simulink model "BFE_TestHarness"  (Simulink 8.6)
settings: Solver=FixedStepDiscrete  StartTime=0.0  StopTime=3  FixedStep=Ts  RelTol=1e-3
PreLoadFcn:
  | addpath('MBD_Tests')
  | 
  | load('Workspace\EnvVar.mat')
  | run('MBD_Tests\MBD_tests_init.m')
  | if exist('tl_preloadfcn','file'), tl_preloadfcn(gcs,402); end
PostLoadFcn:
  | if exist('tl_postloadfcn','file'), tl_postloadfcn(gcs,402); end
InitFcn:
  | if exist('tlds_init','file'), tlds_init(gcs); end
StartFcn:
  | if exist('tlds_start','file'), tlds_start(gcs); end
StopFcn:
  | if exist('tlds_stop','file'), tlds_stop(gcs); end
undefined symbols (not defined in the file): ddv, Ts, u2, u3, u4
libraries: tllib x11, simulink x8, LIB_TF_G_111 x2, LIB_TF_G_12_StepControl x2, LIB_TF_G_112 x1, LIB_TF_G_113 x1
(part 6 of 17)

== system BFE_TestHarness/BFE_AC_BeltFunctionExecution/Subsystem/BFE_AC_BeltFunctionExecution/BFE_AC_BeltFunctionExecution/BFE_runExecuteStandardSteps/ExecuteStandardSteps/SubsystemUpdateConsigns ==
  lMilliOrderIncrement : Inport  RequirementInfo={} %GIDa_5cc21bd3_cc40_44a3_8bbb_1525dfc2aeeb
  lMilliOrder : Inport  RequirementInfo={} %GIDa_1a8363d0_9cc4_4d0f_87bb_7cd28cf3fc20  Port=2
  Add : Sum  RequirementInfo={} %GIDa_7faf4d1b_26d0_400a_863a_5a4ca9203508  SaturateOnIntegerOverflow=on  mask(TL_Sum){data={'output',{'name','s32UpdTargetStepOnGoing','type','Int32','checkmin',1,'checkmax',1},'date',735951.66850537038}}
      settings: CopyFcn=if exist('tl_reset_reviewflag','file')==2,tl_reset_reviewflag(gcbh);end  DeleteFcn=if exist('delete_tlblock','file')==2,delete_tlblock(gcbh);end  NameChangeFcn=if exist('rename_tlblock','file')==2,rename_tlblock(gcbh);end  OpenFcn=if exist('tl_open_blockdlg','file')==2,tl_open_blockdlg(gcbh);else,open_system(gcbh,'parameter');end
      mask Help: eval(['if exist(''tl_online_help'',''file'') == 2, tl_online_help(''Topic'',''TL_Sum''),else, web([''jar:file:///'',matlabroot,''/help/toolbox/simulink/help.jar!/slref/' lower(get_param(gcbh,'Blocktype')) '.html''], ''-helpbrowser''),end'])
      mask Display: plot([-0.05, 1.05, NaN, -0.05, 1.05],[.01, .01, NaN, .99, .99])
  Add1 : Sum  RequirementInfo={} %GIDa_66a69bfa_962f_4ea5_a228_a0bc3a3f5b5e  SaturateOnIntegerOverflow=on  mask(TL_Sum){data={'output',{'name','s32UpdTargetStartStep','type','Int32','checkmin',1,'checkmax',1},'date',735951.66850499995}}
      settings: CopyFcn=if exist('tl_reset_reviewflag','file')==2,tl_reset_reviewflag(gcbh);end  DeleteFcn=if exist('delete_tlblock','file')==2,delete_tlblock(gcbh);end  NameChangeFcn=if exist('rename_tlblock','file')==2,rename_tlblock(gcbh);end  OpenFcn=if exist('tl_open_blockdlg','file')==2,tl_open_blockdlg(gcbh);else,open_system(gcbh,'parameter');end
      mask Help: eval(['if exist(''tl_online_help'',''file'') == 2, tl_online_help(''Topic'',''TL_Sum''),else, web([''jar:file:///'',matlabroot,''/help/toolbox/simulink/help.jar!/slref/' lower(get_param(gcbh,'Blocktype')) '.html''], ''-helpbrowser''),end'])
      mask Display: plot([-0.05, 1.05, NaN, -0.05, 1.05],[.01, .01, NaN, .99, .99])
  SubsystemDetectConsignsChange : Subsystem  RequirementInfo={} %GIDa_913f49ce_43de_40fd_b174_3a8dea1fc7ca
  Switch : Switch  RequirementInfo={} %GIDa_e7269de4_dc33_4d7b_91a9_ffc23af86bd1  Criteria=u2 ~= 0  mask(TL_Switch){data={'output',{'name','s32StepTarget2ms','inheritscaling',1},'threshold',{'scalar',1},'date',735951.66850278934}}
      settings: CopyFcn=if exist('tl_reset_reviewflag','file')==2,tl_reset_reviewflag(gcbh);end  DeleteFcn=if exist('delete_tlblock','file')==2,delete_tlblock(gcbh);end  NameChangeFcn=if exist('rename_tlblock','file')==2,rename_tlblock(gcbh);end  OpenFcn=if exist('tl_open_blockdlg','file')==2,tl_open_blockdlg(gcbh);else,open_system(gcbh,'parameter');end
      mask Help: eval(['if exist(''tl_online_help'',''file'') == 2, tl_online_help(''Topic'',''TL_Switch''),else, web([''jar:file:///'',matlabroot,''/help/toolbox/simulink/help.jar!/slref/' lower(get_param(gcbh,'Blocktype')) '.html''], ''-helpbrowser''),end'])
      mask Display: plot([-0.05, 1.05, NaN, -0.05, 1.05],[.01, .01, NaN, .99, .99])
  Unit Delay : UnitDelay  RequirementInfo={} %GIDa_e30283f1_fb3e_4a2a_b6d4_05ae56e450b9  SampleTime=-1  mask(TL_UnitDelay){data={'output',{'type','Int32'},'state',{'name','s32PrevStepTarget2ms','type','Int32'},'date',735951.66850224533}}
      settings: CopyFcn=if exist('tl_reset_reviewflag','file')==2,tl_reset_reviewflag(gcbh);end  DeleteFcn=if exist('delete_tlblock','file')==2,delete_tlblock(gcbh);end  NameChangeFcn=if exist('rename_tlblock','file')==2,rename_tlblock(gcbh);end  OpenFcn=if exist('tl_open_blockdlg','file')==2,tl_open_blockdlg(gcbh);else,open_system(gcbh,'parameter');end
      mask Help: eval(['if exist(''tl_online_help'',''file'') == 2, tl_online_help(''Topic'',''TL_UnitDelay''),else, web([''jar:file:///'',matlabroot,''/help/toolbox/simulink/help.jar!/slref/' lower(get_param(gcbh,'Blocktype')) '.html''], ''-helpbrowser''),end'])
      mask Display: plot([-0.05, 1.05, NaN, -0.05, 1.05],[.01, .01, NaN, .99, .99])
  bAreConsignsChanged : Outport  RequirementInfo={} %GIDa_218da950_518a_4cec_bd68_380cd2445e8d
  lOrderToApply : Outport  RequirementInfo={} %GIDa_afcc631f_1aa7_4131_a13d_9b5c398a8bc9  Port=2
  wires:
  Add1/1 -> Switch/1
  Unit Delay/1 -> Add/2
  Add/1 -> Switch/3
  Switch/1 -> Unit Delay/1, lOrderToApply/1
  SubsystemDetectConsignsChange/1(bAreConsignsChanged_out) -> bAreConsignsChanged/1, Switch/2
  lMilliOrder/1 -> Add1/1, SubsystemDetectConsignsChange/1(lFirstOrder)
  lMilliOrderIncrement/1 -> Add1/2, Add/1, SubsystemDetectConsignsChange/2(lIncrement)

== system BFE_TestHarness/BFE_AC_BeltFunctionExecution/Subsystem/BFE_AC_BeltFunctionExecution/BFE_AC_BeltFunctionExecution/BFE_runScheduleStep/Critical section for outputs to  protect against ISR access/Switch Case Action Subsystem ==
  In1 : Inport
  Trigger : TriggerPort  TriggerType=function-call
  s32OrderIncrementValue : Outport  PortDimensions=1  mask(TL_Outport){data={'autosar',{'useautosarcommunication',1,'kind',3,'communicationmode',1,'interrunnablevariable','s32OrderIncrementValue'},'date',736809.44014983799}}
      settings: CopyFcn=if exist('tl_reset_reviewflag','file')==2,tl_reset_reviewflag(gcbh);end  DeleteFcn=if exist('delete_tlblock','file')==2,delete_tlblock(gcbh);end  NameChangeFcn=if exist('rename_tlblock','file')==2,rename_tlblock(gcbh);end  OpenFcn=if exist('tl_open_blockdlg','file')==2,tl_open_blockdlg(gcbh);else,open_system(gcbh,'parameter');end
      mask Help: eval(['if exist(''tl_online_help'',''file'') == 2, tl_online_help(''Topic'',''TL_Outport''),else, web([''jar:file:///'',matlabroot,''/help/toolbox/simulink/help.jar!/slref/' lower(get_param(gcbh,'Blocktype')) '.html''], ''-helpbrowser''),end'])
      mask Display: plot([0.2 0.35 NaN 0.65 0.8],[0 1 NaN 0 1]);
  wires:
  In1/1 -> s32OrderIncrementValue/1

== system BFE_TestHarness/BFE_AC_BeltFunctionExecution/Subsystem/BFE_AC_BeltFunctionExecution/BFE_AC_BeltFunctionExecution/BFE_runScheduleStep/Critical section for outputs to  protect against ISR access/Switch Case Action Subsystem1 ==
  In1 : Inport
  Trigger : TriggerPort  TriggerType=function-call
  s32FirstOrderValue : Outport  PortDimensions=1  mask(TL_Outport){data={'autosar',{'useautosarcommunication',1,'kind',3,'communicationmode',1,'interrunnablevariable','s32FirstOrderValue'},'date',736809.44014995371}}
      settings: CopyFcn=if exist('tl_reset_reviewflag','file')==2,tl_reset_reviewflag(gcbh);end  DeleteFcn=if exist('delete_tlblock','file')==2,delete_tlblock(gcbh);end  NameChangeFcn=if exist('rename_tlblock','file')==2,rename_tlblock(gcbh);end  OpenFcn=if exist('tl_open_blockdlg','file')==2,tl_open_blockdlg(gcbh);else,open_system(gcbh,'parameter');end
      mask Help: eval(['if exist(''tl_online_help'',''file'') == 2, tl_online_help(''Topic'',''TL_Outport''),else, web([''jar:file:///'',matlabroot,''/help/toolbox/simulink/help.jar!/slref/' lower(get_param(gcbh,'Blocktype')) '.html''], ''-helpbrowser''),end'])
      mask Display: plot([0.2 0.35 NaN 0.65 0.8],[0 1 NaN 0 1]);
  wires:
  In1/1 -> s32FirstOrderValue/1

== system BFE_TestHarness/BFE_AC_BeltFunctionExecution/Subsystem/BFE_AC_BeltFunctionExecution/BFE_AC_BeltFunctionExecution/BFE_runScheduleStep/Critical section for outputs to  protect against ISR access/Switch Case Action Subsystem2 ==
  In1 : Inport
  Trigger : TriggerPort  TriggerType=function-call
  u16StepDuration : Outport  PortDimensions=1  mask(TL_Outport){data={'autosar',{'useautosarcommunication',1,'kind',3,'communicationmode',1,'interrunnablevariable','u16StepDuration'},'date',736809.44015006942}}
      settings: CopyFcn=if exist('tl_reset_reviewflag','file')==2,tl_reset_reviewflag(gcbh);end  DeleteFcn=if exist('delete_tlblock','file')==2,delete_tlblock(gcbh);end  NameChangeFcn=if exist('rename_tlblock','file')==2,rename_tlblock(gcbh);end  OpenFcn=if exist('tl_open_blockdlg','file')==2,tl_open_blockdlg(gcbh);else,open_system(gcbh,'parameter');end
      mask Help: eval(['if exist(''tl_online_help'',''file'') == 2, tl_online_help(''Topic'',''TL_Outport''),else, web([''jar:file:///'',matlabroot,''/help/toolbox/simulink/help.jar!/slref/' lower(get_param(gcbh,'Blocktype')) '.html''], ''-helpbrowser''),end'])
      mask Display: plot([0.2 0.35 NaN 0.65 0.8],[0 1 NaN 0 1]);
  wires:
  In1/1 -> u16StepDuration/1

== system BFE_TestHarness/BFE_AC_BeltFunctionExecution/Subsystem/BFE_AC_BeltFunctionExecution/BFE_AC_BeltFunctionExecution/BFE_runScheduleStep/Critical section for outputs to  protect against ISR access/Switch Case Action Subsystem3 ==
  In1 : Inport
  Trigger : TriggerPort  TriggerType=function-call
  u8OrderType : Outport  PortDimensions=1  mask(TL_Outport){data={'autosar',{'useautosarcommunication',1,'kind',3,'communicationmode',1,'interrunnablevariable','u8OrderType'},'date',736809.44015030097}}
      settings: CopyFcn=if exist('tl_reset_reviewflag','file')==2,tl_reset_reviewflag(gcbh);end  DeleteFcn=if exist('delete_tlblock','file')==2,delete_tlblock(gcbh);end  NameChangeFcn=if exist('rename_tlblock','file')==2,rename_tlblock(gcbh);end  OpenFcn=if exist('tl_open_blockdlg','file')==2,tl_open_blockdlg(gcbh);else,open_system(gcbh,'parameter');end
      mask Help: eval(['if exist(''tl_online_help'',''file'') == 2, tl_online_help(''Topic'',''TL_Outport''),else, web([''jar:file:///'',matlabroot,''/help/toolbox/simulink/help.jar!/slref/' lower(get_param(gcbh,'Blocktype')) '.html''], ''-helpbrowser''),end'])
      mask Display: plot([0.2 0.35 NaN 0.65 0.8],[0 1 NaN 0 1]);
  wires:
  In1/1 -> u8OrderType/1

== system BFE_TestHarness/BFE_AC_BeltFunctionExecution/Subsystem/BFE_AC_BeltFunctionExecution/BFE_AC_BeltFunctionExecution/ManageRunnables/If Action Subsystem/If Action Subsystem ==
  Action Port : ActionPort  RequirementInfo={} %GIDa_a62ee4e6_0f79_4252_9fe2_412ab995a6fd  ActionType=then
  Function-Call Generator : simulink/Ports & Subsystems/Function-Call Generator  RequirementInfo={} %GIDa_58f86ece_75e2_4389_8d97_59eeed75d555  sample_time=-1  numberOfIterations=1
  Out1 : Outport  RequirementInfo={} %GIDa_7be6b692_a524_497d_b672_83760d64e461
  wires:
  Function-Call Generator/1 -> Out1/1

== system BFE_TestHarness/BFE_AC_BeltFunctionExecution/Subsystem/BFE_AC_BeltFunctionExecution/BFE_AC_BeltFunctionExecution/ManageRunnables/If Action Subsystem1/If Action Subsystem ==
  Action Port : ActionPort  RequirementInfo={} %GIDa_89bb6ac8_18ae_4522_a67e_c5de92d9804a  ActionType=then
  Function-Call Generator : simulink/Ports & Subsystems/Function-Call Generator  RequirementInfo={} %GIDa_4ed9d91c_f3a7_4384_b10d_86c6c5719deb  sample_time=-1  numberOfIterations=1
  Out1 : Outport  RequirementInfo={} %GIDa_e16df5b7_c629_412d_97e3_521d5db63317
  wires:
  Function-Call Generator/1 -> Out1/1

== system BFE_TestHarness/BFE_AC_BeltFunctionExecution/Subsystem/BFE_AC_BeltFunctionExecution/BFE_AC_BeltFunctionExecution/ManageRunnables/If Action Subsystem2/If Action Subsystem1 ==
  Action Port : ActionPort  RequirementInfo={} %GIDa_29c84838_766b_4990_bc41_364801b2a2c1  ActionType=then
  Function-Call Generator : simulink/Ports & Subsystems/Function-Call Generator  RequirementInfo={} %GIDa_00d024fe_ccfb_4152_8998_5dbb5a8dc91c  sample_time=-1  numberOfIterations=1
  Out1 : Outport  RequirementInfo={} %GIDa_21bb2b30_61bd_4376_a26f_0f487527c63e
  wires:
  Function-Call Generator/1 -> Out1/1

== system BFE_TestHarness/BFE_AC_BeltFunctionExecution/Subsystem/BFE_AC_BeltFunctionExecution/BFE_AC_BeltFunctionExecution/ManageRunnables/If Action Subsystem2/If Action Subsystem2 ==
  Action Port : ActionPort  RequirementInfo={} %GIDa_7511eba7_1284_477b_a038_8ef99bfcc2bb  ActionType=else
  Function-Call Generator : simulink/Ports & Subsystems/Function-Call Generator  RequirementInfo={} %GIDa_1326366b_347a_4b1b_b860_6f0899239335  sample_time=-1  numberOfIterations=1
  Out1 : Outport  RequirementInfo={} %GIDa_86f1c9bb_def5_449e_be28_356b79e30475
  wires:
  Function-Call Generator/1 -> Out1/1

== system BFE_TestHarness/BFE_AC_BeltFunctionExecution/Subsystem/BFE_AC_BeltFunctionExecution/BFE_AC_BeltFunctionExecution/ManageRunnables/If Action Subsystem3/If Action Subsystem1 ==
  Action Port : ActionPort  RequirementInfo={} %GIDa_99ef5362_0467_4fc1_9784_994714b2c9a7  ActionType=then
  Function-Call Generator : simulink/Ports & Subsystems/Function-Call Generator  RequirementInfo={} %GIDa_c0aab7a0_dc5d_4927_bcec_735c68472a75  sample_time=-1  numberOfIterations=1
  Out1 : Outport  RequirementInfo={} %GIDa_15a0167e_97c9_4a94_b857_ffa23d77dc58
  wires:
  Function-Call Generator/1 -> Out1/1

== system BFE_TestHarness/BFE_AC_BeltFunctionExecution/Subsystem/BFE_AC_BeltFunctionExecution/BFE_AC_BeltFunctionExecution/BFE_runExecuteHighPowerStep/HP feature activated/CurrentRegulation/BoostInterruptConditions_MotorCurrent ==
  note: If the duty cycle of the PWM for the boost is maximum and if the current is too weak, the boost is interrupted (the value of the duty cycle is decreased)
  s16Current : Inport  RequirementInfo={} %GIDa_fed87945_4a58_47d6_bead_1101b99165da
  s16Integer : Inport  RequirementInfo={} %GIDa_19139cd3_6afd_4d73_a336_46a3cf0ace48  Port=2
  s16IntegerMax : Inport  RequirementInfo={} %GIDa_a1f576fc_1114_4384_8991_b2635a757868  Port=3
  KU8_MIN_CURRENT_DURING_BOOST : Constant  RequirementInfo={} %GIDa_fe38ee79_2149_41c8_8830_b3ef7000511c  Value=ddv('BFE_Config_Data/KU8_MIN_CURRENT_DURING_BOOST')  mask(TL_Constant){data={'output',{'variable','BFE_Config_Data/KU8_MIN_CURRENT_DURING_BOOST'},'date',735951.6685871759}}
      settings: CopyFcn=if exist('tl_reset_reviewflag','file')==2,tl_reset_reviewflag(gcbh);end  DeleteFcn=if exist('delete_tlblock','file')==2,delete_tlblock(gcbh);end  NameChangeFcn=if exist('rename_tlblock','file')==2,rename_tlblock(gcbh);end  OpenFcn=if exist('tl_open_blockdlg','file')==2,tl_open_blockdlg(gcbh);else,open_system(gcbh,'parameter');end
      mask Help: eval(['if exist(''tl_online_help'',''file'') == 2, tl_online_help(''Topic'',''TL_Constant''),else, web([''jar:file:///'',matlabroot,''/help/toolbox/simulink/help.jar!/slref/' lower(get_param(gcbh,'Blocktype')) '.html''], ''-helpbrowser''),end'])
      mask Display: plot([-0.05, 1.05, NaN, -0.05, 1.05],[.01, .01, NaN, .99, .99])
  Logical Operator1 : Logic  RequirementInfo={} %GIDa_242a9706_3112_44f3_83e7_a7f476e04a26  AllPortsSameDT=off  OutDataTypeStr=boolean  mask(TL_LogicalOperator){data={'output',{'name','bBoostInterrupt'},'date',735951.66858680558}}
      settings: DeleteFcn=if exist('delete_tlblock','file')==2,delete_tlblock(gcbh);end  NameChangeFcn=if exist('rename_tlblock','file')==2,rename_tlblock(gcbh);end  OpenFcn=if exist('tl_open_blockdlg','file')==2,tl_open_blockdlg(gcbh);else,open_system(gcbh,'parameter');end
      mask Help: eval(['if exist(''tl_online_help'',''file'') == 2, tl_online_help(''Topic'',''TL_LogicalOperator''),else, web([''jar:file:///'',matlabroot,''/help/toolbox/simulink/help.jar!/slref/' lower(get_param(gcbh,'Blocktype')) '.html''], ''-helpbrowser''),end'])
      mask Display: plot([-0.05, 1.05, NaN, -0.05, 1.05],[.01, .01, NaN, .99, .99])
  Relational Operator : RelationalOperator  RequirementInfo={} %GIDa_2bfdd7ae_5bd4_46be_b807_9ae38a2e5e84  OutDataTypeStr=boolean  mask(TL_RelationalOperator){data={'date',735951.66858653934}}
      settings: DeleteFcn=if exist('delete_tlblock','file')==2,delete_tlblock(gcbh);end  NameChangeFcn=if exist('rename_tlblock','file')==2,rename_tlblock(gcbh);end  OpenFcn=if exist('tl_open_blockdlg','file')==2,tl_open_blockdlg(gcbh);else,open_system(gcbh,'parameter');end
      mask Help: eval(['if exist(''tl_online_help'',''file'') == 2, tl_online_help(''Topic'',''TL_RelationalOperator''),else, web([''jar:file:///'',matlabroot,''/help/toolbox/simulink/help.jar!/slref/' lower(get_param(gcbh,'Blocktype')) '.html''], ''-helpbrowser''),end'])
      mask Display: plot([-0.05, 1.05, NaN, -0.05, 1.05],[.01, .01, NaN, .99, .99])
  Relational Operator1 : RelationalOperator  RequirementInfo={} %GIDa_3d94211e_eea3_4510_ab5c_091b41b511c7  Operator=<  OutDataTypeStr=boolean  mask(TL_RelationalOperator){data={'date',735951.66858628474}}
      settings: DeleteFcn=if exist('delete_tlblock','file')==2,delete_tlblock(gcbh);end  NameChangeFcn=if exist('rename_tlblock','file')==2,rename_tlblock(gcbh);end  OpenFcn=if exist('tl_open_blockdlg','file')==2,tl_open_blockdlg(gcbh);else,open_system(gcbh,'parameter');end
      mask Help: eval(['if exist(''tl_online_help'',''file'') == 2, tl_online_help(''Topic'',''TL_RelationalOperator''),else, web([''jar:file:///'',matlabroot,''/help/toolbox/simulink/help.jar!/slref/' lower(get_param(gcbh,'Blocktype')) '.html''], ''-helpbrowser''),end'])
      mask Display: plot([-0.05, 1.05, NaN, -0.05, 1.05],[.01, .01, NaN, .99, .99])
  bBoostInterrupt : Outport  RequirementInfo={} %GIDa_c813631b_598e_4f6c_b47e_8999c2167893
  wires:
  Relational Operator/1 -> Logical Operator1/2
  KU8_MIN_CURRENT_DURING_BOOST/1 -> Relational Operator1/2
  Relational Operator1/1 -> Logical Operator1/1
  s16Current/1 -> Relational Operator1/1
  s16Integer/1 -> Relational Operator/1
  s16IntegerMax/1 -> Relational Operator/2
  Logical Operator1/1 -> bBoostInterrupt/1

== system BFE_TestHarness/BFE_AC_BeltFunctionExecution/Subsystem/BFE_AC_BeltFunctionExecution/BFE_AC_BeltFunctionExecution/BFE_runExecuteHighPowerStep/HP feature activated/CurrentRegulation/BoostInterruptConditions_Timing ==
  s16OldInteger : Inport  RequirementInfo={} %GIDa_e89f5e19_b5a3_4ada_b2f7_21fc6d90613f
  bBoostTimeElapsed : Inport  RequirementInfo={} %GIDa_225092f2_0ca9_4ed5_8258_126e03d9d686  Port=2
  KUS_PWM_MAX_BTN : Constant  RequirementInfo={} %GIDa_a70c20e3_f31f_4c1c_a99f_96ca4cd62288  Value=ddv('BFE/KS16_PWM_MAX_BTN')  OutDataTypeStr=uint16  mask(TL_Constant){data={'output',{'variable','BFE/KS16_PWM_MAX_BTN'},'date',735951.66858603014}}
      settings: CopyFcn=if exist('tl_reset_reviewflag','file')==2,tl_reset_reviewflag(gcbh);end  DeleteFcn=if exist('delete_tlblock','file')==2,delete_tlblock(gcbh);end  NameChangeFcn=if exist('rename_tlblock','file')==2,rename_tlblock(gcbh);end  OpenFcn=if exist('tl_open_blockdlg','file')==2,tl_open_blockdlg(gcbh);else,open_system(gcbh,'parameter');end
      mask Help: eval(['if exist(''tl_online_help'',''file'') == 2, tl_online_help(''Topic'',''TL_Constant''),else, web([''jar:file:///'',matlabroot,''/help/toolbox/simulink/help.jar!/slref/' lower(get_param(gcbh,'Blocktype')) '.html''], ''-helpbrowser''),end'])
      mask Display: plot([-0.05, 1.05, NaN, -0.05, 1.05],[.01, .01, NaN, .99, .99])
  Logical Operator1 : Logic  RequirementInfo={} %GIDa_9fd42152_b135_49c9_aa59_88d817c1c9ee  AllPortsSameDT=off  OutDataTypeStr=boolean  mask(TL_LogicalOperator){data={'output',{'name','bStartBoostDecrease'},'date',735951.66858567134}}
      settings: DeleteFcn=if exist('delete_tlblock','file')==2,delete_tlblock(gcbh);end  NameChangeFcn=if exist('rename_tlblock','file')==2,rename_tlblock(gcbh);end  OpenFcn=if exist('tl_open_blockdlg','file')==2,tl_open_blockdlg(gcbh);else,open_system(gcbh,'parameter');end
      mask Help: eval(['if exist(''tl_online_help'',''file'') == 2, tl_online_help(''Topic'',''TL_LogicalOperator''),else, web([''jar:file:///'',matlabroot,''/help/toolbox/simulink/help.jar!/slref/' lower(get_param(gcbh,'Blocktype')) '.html''], ''-helpbrowser''),end'])
      mask Display: plot([-0.05, 1.05, NaN, -0.05, 1.05],[.01, .01, NaN, .99, .99])
  Relational Operator : RelationalOperator  RequirementInfo={} %GIDa_0d852afc_57d9_4a42_8a62_1695fcfafa0b  Operator=>  OutDataTypeStr=boolean  mask(TL_RelationalOperator){data={'output',{'name','bBoostOn'},'date',735951.6685854051}}
      settings: DeleteFcn=if exist('delete_tlblock','file')==2,delete_tlblock(gcbh);end  NameChangeFcn=if exist('rename_tlblock','file')==2,rename_tlblock(gcbh);end  OpenFcn=if exist('tl_open_blockdlg','file')==2,tl_open_blockdlg(gcbh);else,open_system(gcbh,'parameter');end
      mask Help: eval(['if exist(''tl_online_help'',''file'') == 2, tl_online_help(''Topic'',''TL_RelationalOperator''),else, web([''jar:file:///'',matlabroot,''/help/toolbox/simulink/help.jar!/slref/' lower(get_param(gcbh,'Blocktype')) '.html''], ''-helpbrowser''),end'])
      mask Display: plot([-0.05, 1.05, NaN, -0.05, 1.05],[.01, .01, NaN, .99, .99])
  bStartBoostDecrease : Outport  RequirementInfo={} %GIDa_daa43caa_cf1f_47eb_8219_5321a27842ad
  wires:
  Logical Operator1/1 -> bStartBoostDecrease/1
  s16OldInteger/1 -> Relational Operator/1
  KUS_PWM_MAX_BTN/1 -> Relational Operator/2
  bBoostTimeElapsed/1 -> Logical Operator1/1
  Relational Operator/1 -> Logical Operator1/2

== system BFE_TestHarness/BFE_AC_BeltFunctionExecution/Subsystem/BFE_AC_BeltFunctionExecution/BFE_AC_BeltFunctionExecution/BFE_runExecuteHighPowerStep/HP feature activated/CurrentRegulation/CalculateIntegerInit ==
  note: IntegerInit = (6400 * Iorder)/KL30
  s16FirstOrderValue : Inport  RequirementInfo={} %GIDa_c817c6f4_52c0_448f_b6ca_a57fed24fcee
  u16BatteryVoltage : Inport  RequirementInfo={} %GIDa_798de003_9265_4dce_9db6_fac1c754e338  Port=2
  KU16_INIT_INTEGER_GAIN_DEN : Constant  Value=ddv('BFE/KU16_INIT_INTEGER_GAIN_DEN')  OutDataTypeStr=uint16  mask(TL_Constant){data={'output',{'variable','BFE/KU16_INIT_INTEGER_GAIN_DEN'},'date',735951.66858512734}}
      settings: CopyFcn=if exist('tl_reset_reviewflag','file')==2,tl_reset_reviewflag(gcbh);end  DeleteFcn=if exist('delete_tlblock','file')==2,delete_tlblock(gcbh);end  NameChangeFcn=if exist('rename_tlblock','file')==2,rename_tlblock(gcbh);end  OpenFcn=if exist('tl_open_blockdlg','file')==2,tl_open_blockdlg(gcbh);else,open_system(gcbh,'parameter');end
      mask Help: eval(['if exist(''tl_online_help'',''file'') == 2, tl_online_help(''Topic'',''TL_Constant''),else, web([''jar:file:///'',matlabroot,''/help/toolbox/simulink/help.jar!/slref/' lower(get_param(gcbh,'Blocktype')) '.html''], ''-helpbrowser''),end'])
      mask Display: plot([-0.05, 1.05, NaN, -0.05, 1.05],[.01, .01, NaN, .99, .99])
  KU16_INIT_INTEGER_GAIN_NOM : Constant  Value=ddv('BFE/KU16_INIT_INTEGER_GAIN_NOM')  OutDataTypeStr=uint16  mask(TL_Constant){data={'output',{'variable','BFE/KU16_INIT_INTEGER_GAIN_NOM'},'date',735951.66858474538}}
      settings: CopyFcn=if exist('tl_reset_reviewflag','file')==2,tl_reset_reviewflag(gcbh);end  DeleteFcn=if exist('delete_tlblock','file')==2,delete_tlblock(gcbh);end  NameChangeFcn=if exist('rename_tlblock','file')==2,rename_tlblock(gcbh);end  OpenFcn=if exist('tl_open_blockdlg','file')==2,tl_open_blockdlg(gcbh);else,open_system(gcbh,'parameter');end
      mask Help: eval(['if exist(''tl_online_help'',''file'') == 2, tl_online_help(''Topic'',''TL_Constant''),else, web([''jar:file:///'',matlabroot,''/help/toolbox/simulink/help.jar!/slref/' lower(get_param(gcbh,'Blocktype')) '.html''], ''-helpbrowser''),end'])
      mask Display: plot([-0.05, 1.05, NaN, -0.05, 1.05],[.01, .01, NaN, .99, .99])
  KUS_PWM_MAX_BTN : Constant  RequirementInfo={} %GIDa_88135799_6637_44ef_a568_3f4a11047fb4  Value=ddv('BFE/KS16_PWM_MAX_BTN')  OutDataTypeStr=uint16  mask(TL_Constant){data={'output',{'variable','BFE/KS16_PWM_MAX_BTN'},'date',735951.66858435189}}
      settings: CopyFcn=if exist('tl_reset_reviewflag','file')==2,tl_reset_reviewflag(gcbh);end  DeleteFcn=if exist('delete_tlblock','file')==2,delete_tlblock(gcbh);end  NameChangeFcn=if exist('rename_tlblock','file')==2,rename_tlblock(gcbh);end  OpenFcn=if exist('tl_open_blockdlg','file')==2,tl_open_blockdlg(gcbh);else,open_system(gcbh,'parameter');end
      mask Help: eval(['if exist(''tl_online_help'',''file'') == 2, tl_online_help(''Topic'',''TL_Constant''),else, web([''jar:file:///'',matlabroot,''/help/toolbox/simulink/help.jar!/slref/' lower(get_param(gcbh,'Blocktype')) '.html''], ''-helpbrowser''),end'])
      mask Display: plot([-0.05, 1.05, NaN, -0.05, 1.05],[.01, .01, NaN, .99, .99])
  Product1 : Product  RequirementInfo={} %GIDa_5e5e27d2_ccc2_478f_b2ba_8d03c9d029d9  Inputs=**  OutDataTypeStr=uint32  RndMeth=Zero  mask(TL_Product){data={'output',{'type','Int32'},'date',735951.66858395829}}
      settings: CopyFcn=if exist('tl_reset_reviewflag','file')==2,tl_reset_reviewflag(gcbh);end  DeleteFcn=if exist('delete_tlblock','file')==2,delete_tlblock(gcbh);end  NameChangeFcn=if exist('rename_tlblock','file')==2,rename_tlblock(gcbh);end  OpenFcn=if exist('tl_open_blockdlg','file')==2,tl_open_blockdlg(gcbh);else,open_system(gcbh,'parameter');end
      mask Help: eval(['if exist(''tl_online_help'',''file'') == 2, tl_online_help(''Topic'',''TL_Product''),else, web([''jar:file:///'',matlabroot,''/help/toolbox/simulink/help.jar!/slref/' lower(get_param(gcbh,'Blocktype')) '.html''], ''-helpbrowser''),end'])
      mask Display: plot([-0.05, 1.05, NaN, -0.05, 1.05],[.01, .01, NaN, .99, .99])
  Product2 : Product  RequirementInfo={} %GIDa_c96c8a8f_b421_4d94_8a8b_1faf2b26a1c7  Inputs=*/  OutDataTypeStr=uint32  RndMeth=Zero  mask(TL_Product){data={'output',{'name','s16IntegerInit','type','UInt32'},'date',735951.66858358798}}
      settings: CopyFcn=if exist('tl_reset_reviewflag','file')==2,tl_reset_reviewflag(gcbh);end  DeleteFcn=if exist('delete_tlblock','file')==2,delete_tlblock(gcbh);end  NameChangeFcn=if exist('rename_tlblock','file')==2,rename_tlblock(gcbh);end  OpenFcn=if exist('tl_open_blockdlg','file')==2,tl_open_blockdlg(gcbh);else,open_system(gcbh,'parameter');end
      mask Help: eval(['if exist(''tl_online_help'',''file'') == 2, tl_online_help(''Topic'',''TL_Product''),else, web([''jar:file:///'',matlabroot,''/help/toolbox/simulink/help.jar!/slref/' lower(get_param(gcbh,'Blocktype')) '.html''], ''-helpbrowser''),end'])
      mask Display: plot([-0.05, 1.05, NaN, -0.05, 1.05],[.01, .01, NaN, .99, .99])
  Product3 : Product  Inputs=**  OutDataTypeStr=uint32  RndMeth=Zero  mask(TL_Product){data={'output',{'type','UInt32'},'date',735951.66858320602}}
      settings: CopyFcn=if exist('tl_reset_reviewflag','file')==2,tl_reset_reviewflag(gcbh);end  DeleteFcn=if exist('delete_tlblock','file')==2,delete_tlblock(gcbh);end  NameChangeFcn=if exist('rename_tlblock','file')==2,rename_tlblock(gcbh);end  OpenFcn=if exist('tl_open_blockdlg','file')==2,tl_open_blockdlg(gcbh);else,open_system(gcbh,'parameter');end
      mask Help: eval(['if exist(''tl_online_help'',''file'') == 2, tl_online_help(''Topic'',''TL_Product''),else, web([''jar:file:///'',matlabroot,''/help/toolbox/simulink/help.jar!/slref/' lower(get_param(gcbh,'Blocktype')) '.html''], ''-helpbrowser''),end'])
      mask Display: plot([-0.05, 1.05, NaN, -0.05, 1.05],[.01, .01, NaN, .99, .99])
  Product4 : Product  Inputs=*/  OutDataTypeStr=int16  RndMeth=Zero  mask(TL_Product){data={'date',735951.66858284723}}
      settings: CopyFcn=if exist('tl_reset_reviewflag','file')==2,tl_reset_reviewflag(gcbh);end  DeleteFcn=if exist('delete_tlblock','file')==2,delete_tlblock(gcbh);end  NameChangeFcn=if exist('rename_tlblock','file')==2,rename_tlblock(gcbh);end  OpenFcn=if exist('tl_open_blockdlg','file')==2,tl_open_blockdlg(gcbh);else,open_system(gcbh,'parameter');end
      mask Help: eval(['if exist(''tl_online_help'',''file'') == 2, tl_online_help(''Topic'',''TL_Product''),else, web([''jar:file:///'',matlabroot,''/help/toolbox/simulink/help.jar!/slref/' lower(get_param(gcbh,'Blocktype')) '.html''], ''-helpbrowser''),end'])
      mask Display: plot([-0.05, 1.05, NaN, -0.05, 1.05],[.01, .01, NaN, .99, .99])
  s16IntegerInit : Outport  RequirementInfo={} %GIDa_8a96fdce_7e82_4479_aa26_86420613cb0b
  wires:
  KUS_PWM_MAX_BTN/1 -> Product1/2
  s16FirstOrderValue/1 -> Product1/1
  Product1/1 -> Product2/1
  u16BatteryVoltage/1 -> Product2/2
  Product2/1 -> Product3/1
  Product3/1 -> Product4/1
  Product4/1 -> s16IntegerInit/1
  KU16_INIT_INTEGER_GAIN_DEN/1 -> Product4/2
  KU16_INIT_INTEGER_GAIN_NOM/1 -> Product3/2

== system BFE_TestHarness/BFE_AC_BeltFunctionExecution/Subsystem/BFE_AC_BeltFunctionExecution/BFE_AC_BeltFunctionExecution/BFE_runExecuteHighPowerStep/HP feature activated/CurrentRegulation/CalculateSintegerMaxInit ==
  note: Limitation of the maximum duty cycle calculated, in order to have a maximum voltage of 40V in the boost
  u16BatteryVoltage : Inport  RequirementInfo={} %GIDa_620a136e_8b12_4ceb_9311_b3af96ea923d
  Constant1 : Constant  RequirementInfo={} %GIDa_1a748155_f034_49fd_bc6b_44a87648d7c4  Value=ddv('BFE_Config_Data/KUS_VBOOST_MAX')  OutDataTypeStr=Inherit: Inherit via back propagation  mask(TL_Constant){data={'output',{'variable','BFE_Config_Data/KUS_VBOOST_MAX'},'date',735951.66858248843}}
      settings: CopyFcn=if exist('tl_reset_reviewflag','file')==2,tl_reset_reviewflag(gcbh);end  DeleteFcn=if exist('delete_tlblock','file')==2,delete_tlblock(gcbh);end  NameChangeFcn=if exist('rename_tlblock','file')==2,rename_tlblock(gcbh);end  OpenFcn=if exist('tl_open_blockdlg','file')==2,tl_open_blockdlg(gcbh);else,open_system(gcbh,'parameter');end
      mask Help: eval(['if exist(''tl_online_help'',''file'') == 2, tl_online_help(''Topic'',''TL_Constant''),else, web([''jar:file:///'',matlabroot,''/help/toolbox/simulink/help.jar!/slref/' lower(get_param(gcbh,'Blocktype')) '.html''], ''-helpbrowser''),end'])
      mask Display: plot([-0.05, 1.05, NaN, -0.05, 1.05],[.01, .01, NaN, .99, .99])
  Constant2 : Constant  RequirementInfo={} %GIDa_0960b975_fb65_49e2_85be_8beb5812d7a5  Value=ddv('BFE/KS16_PWM_MAX_BTN')  OutDataTypeStr=Inherit: Inherit via back propagation  mask(TL_Constant){data={'output',{'variable','BFE/KS16_PWM_MAX_BTN'},'date',735951.66858210647}}
      settings: CopyFcn=if exist('tl_reset_reviewflag','file')==2,tl_reset_reviewflag(gcbh);end  DeleteFcn=if exist('delete_tlblock','file')==2,delete_tlblock(gcbh);end  NameChangeFcn=if exist('rename_tlblock','file')==2,rename_tlblock(gcbh);end  OpenFcn=if exist('tl_open_blockdlg','file')==2,tl_open_blockdlg(gcbh);else,open_system(gcbh,'parameter');end
      mask Help: eval(['if exist(''tl_online_help'',''file'') == 2, tl_online_help(''Topic'',''TL_Constant''),else, web([''jar:file:///'',matlabroot,''/help/toolbox/simulink/help.jar!/slref/' lower(get_param(gcbh,'Blocktype')) '.html''], ''-helpbrowser''),end'])
      mask Display: plot([-0.05, 1.05, NaN, -0.05, 1.05],[.01, .01, NaN, .99, .99])
  KS16_INTEGER_MAX_ABSOLUTE : Constant  Value=ddv('BFE_Config_Data/KS16_INTEGER_MAX_ABSOLUTE')  OutDataTypeStr=int16  mask(TL_Constant){data={'output',{'variable','BFE_Config_Data/KS16_INTEGER_MAX_ABSOLUTE'},'date',735951.66858149308}}
      settings: CopyFcn=if exist('tl_reset_reviewflag','file')==2,tl_reset_reviewflag(gcbh);end  DeleteFcn=if exist('delete_tlblock','file')==2,delete_tlblock(gcbh);end  NameChangeFcn=if exist('rename_tlblock','file')==2,rename_tlblock(gcbh);end  OpenFcn=if exist('tl_open_blockdlg','file')==2,tl_open_blockdlg(gcbh);else,open_system(gcbh,'parameter');end
      mask Help: eval(['if exist(''tl_online_help'',''file'') == 2, tl_online_help(''Topic'',''TL_Constant''),else, web([''jar:file:///'',matlabroot,''/help/toolbox/simulink/help.jar!/slref/' lower(get_param(gcbh,'Blocktype')) '.html''], ''-helpbrowser''),end'])
      mask Display: plot([-0.05, 1.05, NaN, -0.05, 1.05],[.01, .01, NaN, .99, .99])
  Product3 : Product  RequirementInfo={} %GIDa_91f651fb_0754_4e5e_8e9a_6edd4d7f9d1a  Inputs=**  OutDataTypeStr=uint32  RndMeth=Zero  mask(TL_Product){data={'output',{'type','UInt32'},'date',735951.66858108796}}
      settings: CopyFcn=if exist('tl_reset_reviewflag','file')==2,tl_reset_reviewflag(gcbh);end  DeleteFcn=if exist('delete_tlblock','file')==2,delete_tlblock(gcbh);end  NameChangeFcn=if exist('rename_tlblock','file')==2,rename_tlblock(gcbh);end  OpenFcn=if exist('tl_open_blockdlg','file')==2,tl_open_blockdlg(gcbh);else,open_system(gcbh,'parameter');end
      mask Help: eval(['if exist(''tl_online_help'',''file'') == 2, tl_online_help(''Topic'',''TL_Product''),else, web([''jar:file:///'',matlabroot,''/help/toolbox/simulink/help.jar!/slref/' lower(get_param(gcbh,'Blocktype')) '.html''], ''-helpbrowser''),end'])
      mask Display: plot([-0.05, 1.05, NaN, -0.05, 1.05],[.01, .01, NaN, .99, .99])
  Product4 : Product  RequirementInfo={} %GIDa_06fd24dd_57e4_4fa4_b551_3037a26c2614  Inputs=*/  OutDataTypeStr=int16  RndMeth=Zero  mask(TL_Product){data={'output',{'name','s16IntegerMaxInit'},'date',735951.66858064814}}
      settings: CopyFcn=if exist('tl_reset_reviewflag','file')==2,tl_reset_reviewflag(gcbh);end  DeleteFcn=if exist('delete_tlblock','file')==2,delete_tlblock(gcbh);end  NameChangeFcn=if exist('rename_tlblock','file')==2,rename_tlblock(gcbh);end  OpenFcn=if exist('tl_open_blockdlg','file')==2,tl_open_blockdlg(gcbh);else,open_system(gcbh,'parameter');end
      mask Help: eval(['if exist(''tl_online_help'',''file'') == 2, tl_online_help(''Topic'',''TL_Product''),else, web([''jar:file:///'',matlabroot,''/help/toolbox/simulink/help.jar!/slref/' lower(get_param(gcbh,'Blocktype')) '.html''], ''-helpbrowser''),end'])
      mask Display: plot([-0.05, 1.05, NaN, -0.05, 1.05],[.01, .01, NaN, .99, .99])
  Relational Operator : RelationalOperator  Operator=<  OutDataTypeStr=boolean  mask(TL_RelationalOperator){data={'output',{'name','bIsIntegerMaxTooHigh'},'date',735951.66858028935}}
      settings: DeleteFcn=if exist('delete_tlblock','file')==2,delete_tlblock(gcbh);end  NameChangeFcn=if exist('rename_tlblock','file')==2,rename_tlblock(gcbh);end  OpenFcn=if exist('tl_open_blockdlg','file')==2,tl_open_blockdlg(gcbh);else,open_system(gcbh,'parameter');end
      mask Help: eval(['if exist(''tl_online_help'',''file'') == 2, tl_online_help(''Topic'',''TL_RelationalOperator''),else, web([''jar:file:///'',matlabroot,''/help/toolbox/simulink/help.jar!/slref/' lower(get_param(gcbh,'Blocktype')) '.html''], ''-helpbrowser''),end'])
      mask Display: plot([-0.05, 1.05, NaN, -0.05, 1.05],[.01, .01, NaN, .99, .99])
  Scope : Scope  NumInputPorts=4
  Switch : Switch  Criteria=u2 ~= 0  OutDataTypeStr=int16  mask(TL_Switch){data={'output',{'name','s16Integer_MaxInit'},'date',735951.66857998841}}
      settings: CopyFcn=if exist('tl_reset_reviewflag','file')==2,tl_reset_reviewflag(gcbh);end  DeleteFcn=if exist('delete_tlblock','file')==2,delete_tlblock(gcbh);end  NameChangeFcn=if exist('rename_tlblock','file')==2,rename_tlblock(gcbh);end  OpenFcn=if exist('tl_open_blockdlg','file')==2,tl_open_blockdlg(gcbh);else,open_system(gcbh,'parameter');end
      mask Help: eval(['if exist(''tl_online_help'',''file'') == 2, tl_online_help(''Topic'',''TL_Switch''),else, web([''jar:file:///'',matlabroot,''/help/toolbox/simulink/help.jar!/slref/' lower(get_param(gcbh,'Blocktype')) '.html''], ''-helpbrowser''),end'])
      mask Display: plot([-0.05, 1.05, NaN, -0.05, 1.05],[.01, .01, NaN, .99, .99])
  s16IntegerMax : Outport  RequirementInfo={} %GIDa_1379f47d_4640_4b21_a2bd_410fd56b4ca9  InitialOutput=0
  wires:
  Constant1/1 -> Product3/1
  Constant2/1 -> Product3/2
  Product3/1 -> Product4/1
  u16BatteryVoltage/1 -> Product4/2
  Product4/1 -> Scope/3, Switch/1, Relational Operator/1
  Relational Operator/1 -> Scope/2, Switch/2
  Switch/1 -> Scope/1, s16IntegerMax/1
  KS16_INTEGER_MAX_ABSOLUTE/1 -> Scope/4, Relational Operator/2, Switch/3

== system BFE_TestHarness/BFE_AC_BeltFunctionExecution/Subsystem/BFE_AC_BeltFunctionExecution/BFE_AC_BeltFunctionExecution/BFE_runExecuteHighPowerStep/HP feature activated/CurrentRegulation/Calculate_MotorPowerOrder ==
  note: s16MotorPowerOrder = PWM_BTN + PWM_Boost
      |
      | If (s16IntegerError <= 6400) (no boost)
      | PWM_BTN = s16IntegerError
      | PWM_Boost = 0
      |
      | If (s16IntegerError > 6400) (boost)
      | PWM_BTN = 6400 (100% of duty cycle for the PWM on  the BTN)
      | PWM_Boost = 512 - 512 * 6400 / s16IntegerError
  s16IntegerError : Inport  RequirementInfo={} %GIDa_500d1f7f_8b44_43ff_96c7_2b8a364e049a
  0 : Constant  RequirementInfo={} %GIDa_50f7787c_342a_4440_a967_c53c4a8ed2ff  Value=ddv('Common/KU16_ZERO')  OutDataTypeStr=uint16  mask(TL_Constant){data={'output',{'variable','Common/KU16_ZERO'},'date',735951.66857947921}}
      settings: CopyFcn=if exist('tl_reset_reviewflag','file')==2,tl_reset_reviewflag(gcbh);end  DeleteFcn=if exist('delete_tlblock','file')==2,delete_tlblock(gcbh);end  NameChangeFcn=if exist('rename_tlblock','file')==2,rename_tlblock(gcbh);end  OpenFcn=if exist('tl_open_blockdlg','file')==2,tl_open_blockdlg(gcbh);else,open_system(gcbh,'parameter');end
      mask Help: eval(['if exist(''tl_online_help'',''file'') == 2, tl_online_help(''Topic'',''TL_Constant''),else, web([''jar:file:///'',matlabroot,''/help/toolbox/simulink/help.jar!/slref/' lower(get_param(gcbh,'Blocktype')) '.html''], ''-helpbrowser''),end'])
      mask Display: plot([-0.05, 1.05, NaN, -0.05, 1.05],[.01, .01, NaN, .99, .99])
  KUS_PWM_MAX_BOOST : Constant  RequirementInfo={} %GIDa_0dbe01bf_df81_46b9_bd85_d01ff0081cad  Value=ddv('BFE/KUS_PWM_MAX_BOOST')  OutDataTypeStr=uint16  mask(TL_Constant){data={'output',{'variable','BFE/KUS_PWM_MAX_BOOST'},'date',735951.66857908561}}
      settings: CopyFcn=if exist('tl_reset_reviewflag','file')==2,tl_reset_reviewflag(gcbh);end  DeleteFcn=if exist('delete_tlblock','file')==2,delete_tlblock(gcbh);end  NameChangeFcn=if exist('rename_tlblock','file')==2,rename_tlblock(gcbh);end  OpenFcn=if exist('tl_open_blockdlg','file')==2,tl_open_blockdlg(gcbh);else,open_system(gcbh,'parameter');end
      mask Help: eval(['if exist(''tl_online_help'',''file'') == 2, tl_online_help(''Topic'',''TL_Constant''),else, web([''jar:file:///'',matlabroot,''/help/toolbox/simulink/help.jar!/slref/' lower(get_param(gcbh,'Blocktype')) '.html''], ''-helpbrowser''),end'])
      mask Display: plot([-0.05, 1.05, NaN, -0.05, 1.05],[.01, .01, NaN, .99, .99])
  KUS_PWM_MAX_BTN : Constant  RequirementInfo={} %GIDa_6f58d92d_9305_461c_b539_4e45f4acd860  Value=ddv('BFE/KS16_PWM_MAX_BTN')  OutDataTypeStr=uint16  mask(TL_Constant){data={'output',{'variable','BFE/KS16_PWM_MAX_BTN'},'date',735951.6685786806}}
      settings: CopyFcn=if exist('tl_reset_reviewflag','file')==2,tl_reset_reviewflag(gcbh);end  DeleteFcn=if exist('delete_tlblock','file')==2,delete_tlblock(gcbh);end  NameChangeFcn=if exist('rename_tlblock','file')==2,rename_tlblock(gcbh);end  OpenFcn=if exist('tl_open_blockdlg','file')==2,tl_open_blockdlg(gcbh);else,open_system(gcbh,'parameter');end
      mask Help: eval(['if exist(''tl_online_help'',''file'') == 2, tl_online_help(''Topic'',''TL_Constant''),else, web([''jar:file:///'',matlabroot,''/help/toolbox/simulink/help.jar!/slref/' lower(get_param(gcbh,'Blocktype')) '.html''], ''-helpbrowser''),end'])
      mask Display: plot([-0.05, 1.05, NaN, -0.05, 1.05],[.01, .01, NaN, .99, .99])
  Product : Product  RequirementInfo={} %GIDa_668fa4a2_5714_407c_85e4_1f12b9212566  Inputs=**  RndMeth=Zero  mask(TL_Product){data={'output',{'type','Int32'},'date',735951.668578287}}
      settings: CopyFcn=if exist('tl_reset_reviewflag','file')==2,tl_reset_reviewflag(gcbh);end  DeleteFcn=if exist('delete_tlblock','file')==2,delete_tlblock(gcbh);end  NameChangeFcn=if exist('rename_tlblock','file')==2,rename_tlblock(gcbh);end  OpenFcn=if exist('tl_open_blockdlg','file')==2,tl_open_blockdlg(gcbh);else,open_system(gcbh,'parameter');end
      mask Help: eval(['if exist(''tl_online_help'',''file'') == 2, tl_online_help(''Topic'',''TL_Product''),else, web([''jar:file:///'',matlabroot,''/help/toolbox/simulink/help.jar!/slref/' lower(get_param(gcbh,'Blocktype')) '.html''], ''-helpbrowser''),end'])
      mask Display: plot([-0.05, 1.05, NaN, -0.05, 1.05],[.01, .01, NaN, .99, .99])
  Product1 : Product  RequirementInfo={} %GIDa_cf56e999_4331_4f0c_bf0d_f732e6fbd690  Inputs=/*  RndMeth=Zero  mask(TL_Product){data={'output',{'name','s16BoostDuty'},'date',735951.66857789352}}
      settings: CopyFcn=if exist('tl_reset_reviewflag','file')==2,tl_reset_reviewflag(gcbh);end  DeleteFcn=if exist('delete_tlblock','file')==2,delete_tlblock(gcbh);end  NameChangeFcn=if exist('rename_tlblock','file')==2,rename_tlblock(gcbh);end  OpenFcn=if exist('tl_open_blockdlg','file')==2,tl_open_blockdlg(gcbh);else,open_system(gcbh,'parameter');end
      mask Help: eval(['if exist(''tl_online_help'',''file'') == 2, tl_online_help(''Topic'',''TL_Product''),else, web([''jar:file:///'',matlabroot,''/help/toolbox/simulink/help.jar!/slref/' lower(get_param(gcbh,'Blocktype')) '.html''], ''-helpbrowser''),end'])
      mask Display: plot([-0.05, 1.05, NaN, -0.05, 1.05],[.01, .01, NaN, .99, .99])
  Relational Operator : RelationalOperator  RequirementInfo={} %GIDa_f2863f72_9f7c_4caa_9ce4_949b80a18da1  Operator=<  OutDataTypeStr=boolean  mask(TL_RelationalOperator){data={'output',{'name','bIsBoostNeeded'},'date',735951.6685775232}}
      settings: DeleteFcn=if exist('delete_tlblock','file')==2,delete_tlblock(gcbh);end  NameChangeFcn=if exist('rename_tlblock','file')==2,rename_tlblock(gcbh);end  OpenFcn=if exist('tl_open_blockdlg','file')==2,tl_open_blockdlg(gcbh);else,open_system(gcbh,'parameter');end
      mask Help: eval(['if exist(''tl_online_help'',''file'') == 2, tl_online_help(''Topic'',''TL_RelationalOperator''),else, web([''jar:file:///'',matlabroot,''/help/toolbox/simulink/help.jar!/slref/' lower(get_param(gcbh,'Blocktype')) '.html''], ''-helpbrowser''),end'])
      mask Display: plot([-0.05, 1.05, NaN, -0.05, 1.05],[.01, .01, NaN, .99, .99])
  Sum : Sum  RequirementInfo={} %GIDa_df464ff4_6cdf_4609_8486_f438d06fea7c  Inputs=-+  OutDataTypeStr=int16  mask(TL_Sum){data={'output',{'type','UInt16'},'date',735951.6685772338}}
      settings: CopyFcn=if exist('tl_reset_reviewflag','file')==2,tl_reset_reviewflag(gcbh);end  DeleteFcn=if exist('delete_tlblock','file')==2,delete_tlblock(gcbh);end  NameChangeFcn=if exist('rename_tlblock','file')==2,rename_tlblock(gcbh);end  OpenFcn=if exist('tl_open_blockdlg','file')==2,tl_open_blockdlg(gcbh);else,open_system(gcbh,'parameter');end
      mask Help: eval(['if exist(''tl_online_help'',''file'') == 2, tl_online_help(''Topic'',''TL_Sum''),else, web([''jar:file:///'',matlabroot,''/help/toolbox/simulink/help.jar!/slref/' lower(get_param(gcbh,'Blocktype')) '.html''], ''-helpbrowser''),end'])
      mask Display: plot([-0.05, 1.05, NaN, -0.05, 1.05],[.01, .01, NaN, .99, .99])
  Switch : Switch  RequirementInfo={} %GIDa_204d81c4_87ce_4ee2_9c98_7a54fedd0c97  Criteria=u2 ~= 0  OutDataTypeStr=int16  mask(TL_Switch){data={'output',{'name','s16PWMOrderHB','class','DISP_LOCAL'},'date',735951.66857682867}}
      settings: CopyFcn=if exist('tl_reset_reviewflag','file')==2,tl_reset_reviewflag(gcbh);end  DeleteFcn=if exist('delete_tlblock','file')==2,delete_tlblock(gcbh);end  NameChangeFcn=if exist('rename_tlblock','file')==2,rename_tlblock(gcbh);end  OpenFcn=if exist('tl_open_blockdlg','file')==2,tl_open_blockdlg(gcbh);else,open_system(gcbh,'parameter');end
      mask Help: eval(['if exist(''tl_online_help'',''file'') == 2, tl_online_help(''Topic'',''TL_Switch''),else, web([''jar:file:///'',matlabroot,''/help/toolbox/simulink/help.jar!/slref/' lower(get_param(gcbh,'Blocktype')) '.html''], ''-helpbrowser''),end'])
      mask Display: plot([-0.05, 1.05, NaN, -0.05, 1.05],[.01, .01, NaN, .99, .99])
  Switch1 : Switch  RequirementInfo={} %GIDa_988c73b0_26c1_47d6_af6f_1e639ec65949  Criteria=u2 ~= 0  mask(TL_Switch){data={'output',{'name','u16PWMOrderBoost','class','DISP_LOCAL','type','UInt16'},'date',735951.66857626161}}
      settings: CopyFcn=if exist('tl_reset_reviewflag','file')==2,tl_reset_reviewflag(gcbh);end  DeleteFcn=if exist('delete_tlblock','file')==2,delete_tlblock(gcbh);end  NameChangeFcn=if exist('rename_tlblock','file')==2,rename_tlblock(gcbh);end  OpenFcn=if exist('tl_open_blockdlg','file')==2,tl_open_blockdlg(gcbh);else,open_system(gcbh,'parameter');end
      mask Help: eval(['if exist(''tl_online_help'',''file'') == 2, tl_online_help(''Topic'',''TL_Switch''),else, web([''jar:file:///'',matlabroot,''/help/toolbox/simulink/help.jar!/slref/' lower(get_param(gcbh,'Blocktype')) '.html''], ''-helpbrowser''),end'])
      mask Display: plot([-0.05, 1.05, NaN, -0.05, 1.05],[.01, .01, NaN, .99, .99])
  s16DutyCycle_HB : Outport  RequirementInfo={} %GIDa_58dc8d84_d465_4ab7_84f8_a38dfb74c676
  u16DutyCycle_Boost : Outport  RequirementInfo={} %GIDa_2aafbd65_36ce_419a_a377_4732f2ea4b13  Port=2
  wires:
  KUS_PWM_MAX_BTN/1 -> Product/1, Relational Operator/2, Switch/3
  s16IntegerError/1 -> Switch/1, Product1/1, Relational Operator/1
  Product/1 -> Product1/2
  Relational Operator/1 -> Switch/2, Switch1/2
  Switch/1 -> s16DutyCycle_HB/1
  KUS_PWM_MAX_BOOST/1 -> Product/2, Sum/2
  Product1/1 -> Sum/1
  Sum/1 -> Switch1/3
  Switch1/1 -> u16DutyCycle_Boost/1
  0/1 -> Switch1/1
